simulink model "BLDC_Speed_Torque_Current_ClosedLoop"  (R2022b)
settings: Solver=ode4  StartTime=0.0  StopTime=3  FixedStep=1e-6  RelTol=1e-3
model workspace (MAT data in the model file):
  Ctrol_Mode = 4
  Current_Control_Mode = 2
  Current_PID_Upper_Limit = 1
  PWM_Period = 0.0001
  Speed_I = 10
  Speed_P = 10
  Speed_PID_Upper_Limit = 0.02
  Ts_time = 1e-06
  current_I = 10
  current_P = 100
undefined symbols (not defined in the file): DiscIntNeverNeededParam, sigbuilder_block
libraries: simulink x18, slpidlib x6, dsparch4 x3, eePwmGenerator x3, spsSeriesRLCBranchLib x2, spsPermanentMagnetSynchronousMachineLib x1, spsCurrentMeasurementLib x1, spsDCVoltageSourceLib x1, slctrlblks x1, spsTwoLevelConverterLib x1, spspowerguiLib x1
(part 1 of 2)
settings Model: Creator=31904  LastModifiedBy=31904

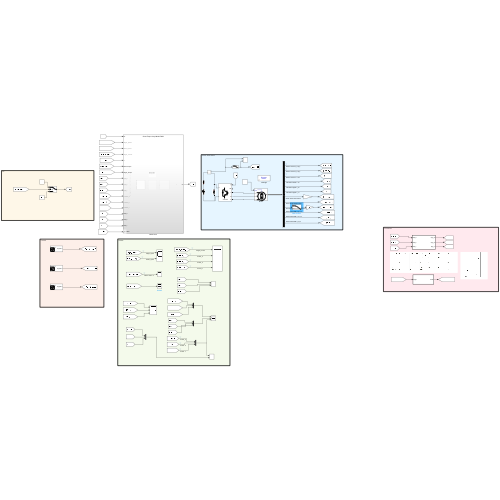
[thumbnail: Simulink's stored preview of the top-level diagram]
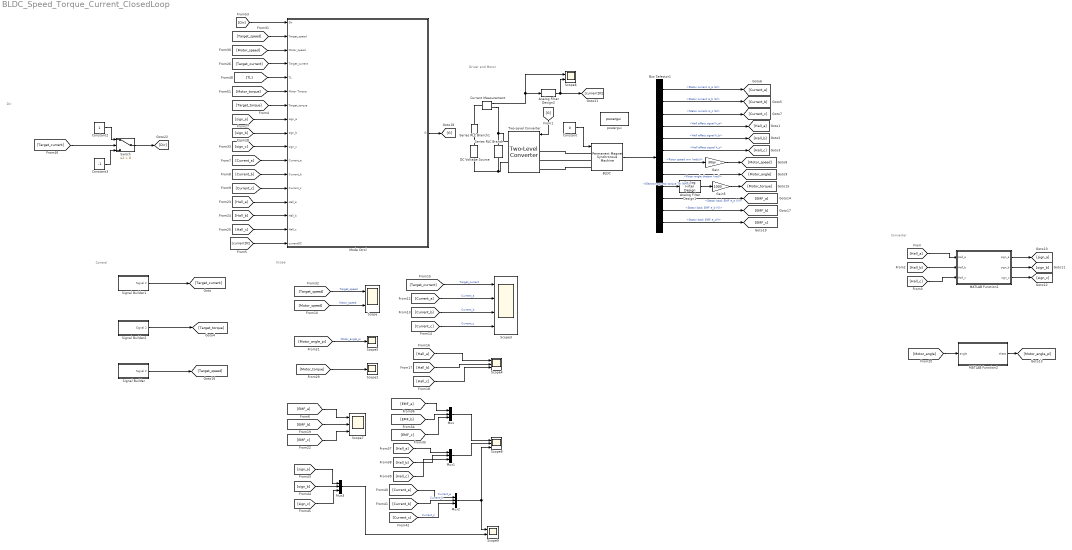
== system BLDC_Speed_Torque_Current_ClosedLoop ==
  note: Dir
  note: Converter
  note: Control
  note: Scope
  note: Driver and Motor
  Analog Filter Design1 : dsparch4/Analog Filter Design  method=Butterworth  filttype=Lowpass  N=1  Wlo=1e2  Whi=80  Rp=2  Rs=40
  Analog Filter Design2 : dsparch4/Analog Filter Design  method=Butterworth  filttype=Lowpass  N=1  Wlo=100  Whi=80  Rp=2  Rs=40
  BLDC : spsPermanentMagnetSynchronousMachineLib/Permanent Magnet Synchronous Machine  NbPhases=3  FluxDistribution=Trapezoidal  RotorType=Round  MechanicalLoad=Torque Tm  PresetModel=No  ShowDetailedParameters=on  MeasurementBus=off  Resistance=1.005  Inductance=66e-6  dqInductances=[8.5e-3,8.5e-3]  La=0.0004  MachineConstant=Torque Constant (N.m / A_peak)  Flux=0.00785  VoltageCst=3.2882  TorqueCst=0.0314  Flat=120  Mechanical=[3e-05 0 2 0]  PolePairs=4  InitialConditions=[0,0, 0,0]  InitialConditions5ph=[0 0 0 0 0 0]  RefAngle=Aligned with phase A axis (original Park)  IterativeDiscreteModel=Trapezoidal non iterative  TsBlock=-1  TsPowergui=0
  Bus Selector1 : BusSelector  OutputSignals=Stator current is_a (A),Stator current is_b (A),Stator current is_c (A),Hall effect signal h_a,Hall effect signal h_b,Hall effect signal h_c,Rotor speed wm (rad/s),Rotor angle thetam (rad),Electromagnetic torque Te (N*m),Stator back EMF e_a (V),Stator back EMF e_b (V),Stator back EMF e_cV)
  Constant : Constant  Value=0
  Constant2 : Constant
  Constant3 : Constant  Value=-1
  Current Measurement : spsCurrentMeasurementLib/Current Measurement  PhasorSimulation=off  OutputType=Complex  PSBequivalent=0
  DC Voltage Source : spsDCVoltageSourceLib/DC Voltage Source  Amplitude=28  Measurements=None
  Gain : Gain  Gain=30/pi
  Gain5 : Gain  Gain=1000
  MATLAB Function1 : MATLAB Function  TreatAsAtomicUnit=on
  MATLAB Function2 : MATLAB Function  TreatAsAtomicUnit=on
  Mode Ctrol : Subsystem  Variant=on
  Mux{,1..3} (4 alike) : Mux  Inputs=3
  Scope : Scope  NumInputPorts=2
  Scope2 : Scope
  Scope3 : Scope  NumInputPorts=4
  Scope4 : Scope  NumInputPorts=3
  Scope5 : Scope
  Scope6 : Scope  NumInputPorts=2
  Scope7 : Scope  NumInputPorts=3
  Scope8 : Scope  NumInputPorts=3
  Scope9 : Scope  NumInputPorts=2
  Series RLC Branch : spsSeriesRLCBranchLib/Series RLC Branch  LConnTagsString=__new0  RConnTagsString=__new0  BranchType=C  Resistance=1  Inductance=1e-3  SetiL0=off  InitialCurrent=0  Capacitance=1e-6  Setx0=off  InitialVoltage=0  Measurements=None
  Series RLC Branch1 : spsSeriesRLCBranchLib/Series RLC Branch  LConnTagsString=__new0  RConnTagsString=__new0  BranchType=R  Resistance=1  Inductance=1e-3  SetiL0=off  InitialCurrent=0  Capacitance=1e-6  Setx0=off  InitialVoltage=0  Measurements=None
  Signal Builder : Subsystem  Tag=STV Subsys  LoadFcn=sigbuilder_block('load');  StartFcn=sigbuilder_block('start');  StopFcn=sigbuilder_block('stop');  ClipboardFcn=sigbuilder_block('clipboard');  mask(Sigbuilder block){tuvar=[0:10]}
      mask help: Simulink:masks:SigbuilderBlock_MD
      mask init:
      | if ~strcmp(get_param(bdroot(gcbh),'SimulationStatus'),'stopped') tuvar = sigbuilder_block('maskInit'); end
      settings: CopyFcn=sigbuilder_block('copy');  DeleteFcn=sigbuilder_block('delete');  ModelCloseFcn=sigbuilder_block('modelClose');  PreSaveFcn=sigbuilder_block('preSave');  PauseFcn=sigbuilder_block('pause');  ContinueFcn=sigbuilder_block('continue');  NameChangeFcn=sigbuilder_block('namechange');  OpenFcn=sigbuilder_block('open',[281.4 79.2 550.8 400.2 ]);  CloseFcn=sigbuilder_block('close');
      mask Display: plot(0, 0, 100, 100,[2, 2, 32, 32, 2], [68, 8, 8, 68, 68],[32, 2], [38, 38], [32, 19, 2],[53, 60, 44], [32, 17, 17, 2],[16, 16, 31, 31]);txt = getActiveGroup(gcbh);text(2, 100, txt,'verticalAlignment', 'top');
  Signal Builder1 : Subsystem  Tag=STV Subsys  LoadFcn=sigbuilder_block('load');  StartFcn=sigbuilder_block('start');  StopFcn=sigbuilder_block('stop');  ClipboardFcn=sigbuilder_block('clipboard');  mask(Sigbuilder block){tuvar=[0:10]}
      mask help: Simulink:masks:SigbuilderBlock_MD
      mask init:
      | if ~strcmp(get_param(bdroot(gcbh),'SimulationStatus'),'stopped') tuvar = sigbuilder_block('maskInit'); end
      settings: CopyFcn=sigbuilder_block('copy');  DeleteFcn=sigbuilder_block('delete');  ModelCloseFcn=sigbuilder_block('modelClose');  PreSaveFcn=sigbuilder_block('preSave');  PauseFcn=sigbuilder_block('pause');  ContinueFcn=sigbuilder_block('continue');  NameChangeFcn=sigbuilder_block('namechange');  OpenFcn=sigbuilder_block('open',[5.4 30 1141.2 523.8 ]);  CloseFcn=sigbuilder_block('close');
      mask Display: plot(0, 0, 100, 100,[2, 2, 32, 32, 2], [68, 8, 8, 68, 68],[32, 2], [38, 38], [32, 19, 2],[53, 60, 44], [32, 17, 17, 2],[16, 16, 31, 31]);txt = getActiveGroup(gcbh);text(2, 100, txt,'verticalAlignment', 'top');
  Signal Builder2 : Subsystem  Tag=STV Subsys  LoadFcn=sigbuilder_block('load');  StartFcn=sigbuilder_block('start');  StopFcn=sigbuilder_block('stop');  ClipboardFcn=sigbuilder_block('clipboard');  mask(Sigbuilder block){tuvar=[0:10]}
      mask help: Simulink:masks:SigbuilderBlock_MD
      mask init:
      | if ~strcmp(get_param(bdroot(gcbh),'SimulationStatus'),'stopped') tuvar = sigbuilder_block('maskInit'); end
      settings: CopyFcn=sigbuilder_block('copy');  DeleteFcn=sigbuilder_block('delete');  ModelCloseFcn=sigbuilder_block('modelClose');  PreSaveFcn=sigbuilder_block('preSave');  PauseFcn=sigbuilder_block('pause');  ContinueFcn=sigbuilder_block('continue');  NameChangeFcn=sigbuilder_block('namechange');  OpenFcn=sigbuilder_block('open',[281.4 79.2 550.8 400.2 ]);  CloseFcn=sigbuilder_block('close');
      mask Display: plot(0, 0, 100, 100,[2, 2, 32, 32, 2], [68, 8, 8, 68, 68],[32, 2], [38, 38], [32, 19, 2],[53, 60, 44], [32, 17, 17, 2],[16, 16, 31, 31]);txt = getActiveGroup(gcbh);text(2, 100, txt,'verticalAlignment', 'top');
  Switch : Switch  Criteria=u2 > Threshold  SaturateOnIntegerOverflow=off  InputSameDT=off
  Two-Level Converter : spsTwoLevelConverterLib/Two-Level Converter  ModelType=Switching devices  Ron=0.0001  Rs=1e6  Cs=inf  Vforward=[0,0]  Ron_Diode=1e-3  Rs_Diode=1e6  Cs_Diode=inf  Vf_Diode=1e-3  Rs_CurrentSource=inf  Ron_ACsource=1e-3
  powergui : spspowerguiLib/powergui  Priority=1  SimulationMode=Discrete  SampleTime=0.000001  frequency=60  Iterations=50  frequencyindice=0  Pbase=100e6  ErrMax=1e-4  UnitsV=kV  UnitsW=MW  buscounter=0  FunctionMessages=off  echomessages=off  EnableUseOfTLC=off  CurrentSourceSwitches=off  DisableSnubberDevices=off  DisableRonSwitches=off  DisableVfSwitches=off  DisplayEquations=off  AutomaticDiscreteSolvers=off  SolverType=Tustin/Backward Euler (TBE)  Interpol=off  ExternalGateDelay=off  methode=off  Ts=100  x0status=blocks  SPID=on  SwTol=0  HookPort=off  NonlinearTolerance=1e-4  nMaxIteration=100  ContinueOnMaxIteration=off  RestoreLinks=warning  ResistiveCurrentMeasurement=off  Frange=[0:2:500]  Ylog=off  Xlog=on  ShowGrid=off  save=off  variable=ZData  structure=0  ZoomFFT=off  StartTime=0.0  cycles=1  DisplayStyle=1  fundamental=60  FreqAxis=off  MaxFrequency=1000  frequencyindicesteady=1  RmsSteady=1  display=off
  wires:
  [G] -> Two-Level Converter/1
  Bus Selector1/3 -> [Current_c]  "<Stator current is_c (A)>"
  Bus Selector1/8 -> [Motor_angle]  "<Rotor angle thetam (rad)>"
  Bus Selector1/1 -> [Current_a]  "<Stator current is_a (A)>"
  Bus Selector1/6 -> [Hall_c]  "<Hall effect signal h_c>"
  Bus Selector1/4 -> [Hall_a]  "<Hall effect signal h_a>"
  Bus Selector1/2 -> [Current_b]  "<Stator current is_b (A)>"
  Bus Selector1/7 -> Gain/1  "<Rotor speed wm (rad/s)>"
  Bus Selector1/5 -> [Hall_b]  "<Hall effect signal h_b>"
  [Hall_a] -> MATLAB Function1/1(Hall_a)
  [Hall_b] -> MATLAB Function1/2(Hall_b)
  [Hall_c] -> MATLAB Function1/3(Hall_c)
  MATLAB Function1/1(sign_a) -> [sign_a]
  MATLAB Function1/2(sign_b) -> [sign_b]
  MATLAB Function1/3(sign_c) -> [sign_c]
  [Motor_speed] -> Scope/2  "Motor_speed"
  [Current_a] -> Scope3/2  "Current_a"
  [Current_b] -> Scope3/3  "Current_b"
  [Current_c] -> Scope3/4  "Current_c"
  [Target_current] -> Scope3/1  "Target_current"
  [Hall_a] -> Scope4/1
  [Hall_b] -> Scope4/2
  [Hall_c] -> Scope4/3
  [Motor_angle] -> MATLAB Function2/1(angle)
  [Motor_angle_pi] -> Scope5/1  "Motor_angle_pi"
  MATLAB Function2/1(theta) -> [Motor_angle_pi]
  Bus Selector1/9 -> Analog Filter Design1/1  "<Electromagnetic torque Te (N*m)>"
  [Motor_torque] -> Scope2/1
  [Target_speed] -> Scope/1  "Target_speed"
  Mode Ctrol/1(G) -> [G]
  [sign_a] -> Mode Ctrol/8(sign_a)
  [sign_b] -> Mode Ctrol/9(sign_b)
  [sign_c] -> Mode Ctrol/10(sign_c)
  [Target_current] -> Mode Ctrol/4(Target_current)
  [Target_speed] -> Mode Ctrol/2(Target_speed)
  [Motor_speed] -> Mode Ctrol/3(Motor_speed)
  [Target_torque] -> Mode Ctrol/7(Target_torque)
  [Current_a] -> Mode Ctrol/11(Current_a)
  [Current_b] -> Mode Ctrol/12(Current_b)
  [Current_c] -> Mode Ctrol/13(Current_c)
  Gain/1 -> [Motor_speed]
  Bus Selector1/10 -> [EMF_a]  "<Stator back EMF e_a (V)>"
  Bus Selector1/11 -> [EMF_b]  "<Stator back EMF e_b (V)>"
  Bus Selector1/12 -> [EMF_c]  "<Stator back EMF e_cV)>"
  [EMF_a] -> Scope7/1
  [EMF_b] -> Scope7/2
  [EMF_c] -> Scope7/3
  [Hall_a] -> Mode Ctrol/14(Hall_a)
  [Hall_b] -> Mode Ctrol/15(Hall_b)
  [Hall_c] -> Mode Ctrol/16(Hall_c)
  [EMF_a] -> Mux/1
  [EMF_b] -> Mux/2
  [EMF_c] -> Mux/3
  [Hall_a] -> Mux1/1
  [Hall_b] -> Mux1/2
  [Hall_c] -> Mux1/3
  Mux1/1 -> Scope8/2
  [Current_a] -> Mux2/1  "Current_a"
  [Current_b] -> Mux2/2  "Current_b"
  [Current_c] -> Mux2/3  "Current_c"
  Mux/1 -> Scope8/1
  Mux2/1 -> Scope8/3, Scope9/1
  [sign_a] -> Mux3/1
  [sign_b] -> Mux3/2
  [sign_c] -> Mux3/3
  Mux3/1 -> Scope9/2
  BLDC/1 -> Bus Selector1/1
  [TL] -> Mode Ctrol/5(TL)
  [Motor_torque] -> Mode Ctrol/6(Motor Torque)
  Constant2/1 -> Switch/1
  Constant3/1 -> Switch/3
  Switch/1 -> [Dir]
  [Dir] -> Mode Ctrol/1(Dir)
  Gain5/1 -> [Motor_torque]
  Signal Builder/1(Signal 2) -> [Target_speed]
  Constant/1 -> BLDC/1
  Current Measurement/1 -> Scope6/1, Analog Filter Design2/1
  Analog Filter Design2/1 -> [currentDC], Scope6/2
  [currentDC] -> Mode Ctrol/17(currentDC)
  [Target_current] -> Switch/2
  Signal Builder2/1(Signal 2) -> [Target_torque]
  Signal Builder1/1(Signal 2) -> [Target_current]
  Analog Filter Design1/1 -> Gain5/1
  connections:
  DC Voltage Source/LConn1 -- Two-Level Converter/RConn2 -- Series RLC Branch/RConn1
  BLDC/LConn1 -- Two-Level Converter/LConn1
  BLDC/LConn2 -- Two-Level Converter/LConn2
  BLDC/LConn3 -- Two-Level Converter/LConn3
  Current Measurement/RConn1 -- Two-Level Converter/RConn1 -- Series RLC Branch/LConn1
  Series RLC Branch1/LConn1 -- DC Voltage Source/RConn1
  Series RLC Branch1/RConn1 -- Current Measurement/LConn1

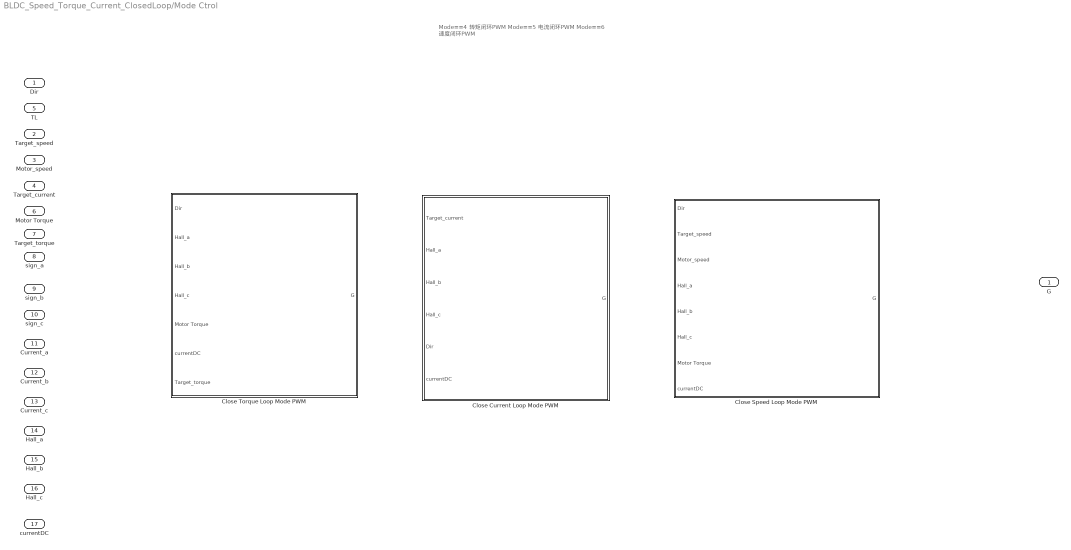
== system BLDC_Speed_Torque_Current_ClosedLoop/Mode Ctrol ==
  note: Mode==4 转矩闭环PWM
      | Mode==5 电流闭环PWM
      | Mode==6 速度闭环PWM
  Dir : Inport
  Target_speed : Inport  Port=2
  Motor_speed : Inport  Port=3
  Target_current : Inport  Port=4
  TL : Inport  Port=5
  Motor Torque : Inport  Port=6
  Target_torque : Inport  Port=7
  sign_a : Inport  Port=8
  sign_b : Inport  Port=9
  sign_c : Inport  Port=10
  Current_a : Inport  Port=11
  Current_b : Inport  Port=12
  Current_c : Inport  Port=13
  Hall_a : Inport  Port=14
  Hall_b : Inport  Port=15
  Hall_c : Inport  Port=16
  currentDC : Inport  Port=17
  Close Current Loop Mode PWM : Subsystem  TreatAsAtomicUnit=on  VariantControl=Ctrol_Mode==5
  Close Speed Loop Mode PWM : Subsystem  TreatAsAtomicUnit=on  VariantControl=Ctrol_Mode==6
  Close Torque Loop Mode PWM : Subsystem  TreatAsAtomicUnit=on  VariantControl=Ctrol_Mode==4
  G : Outport

== system BLDC_Speed_Torque_Current_ClosedLoop/Signal Builder ==
  Demux : Demux  Tag=STV Demux  Outputs=1
      settings: DisplayOption=none
  FromWs : FromWorkspace  Tag=STV FromWs  VariableName=tuvar
      SigBuilderData=|
      | common.afterFinalStr = 'Extrapolate'
      | common.sampleTime = 0
      | dataSet.timeRange = [0 10]
      | dataSet.name = 'Group 1'
      | sbobj.Groups.Name = 'Group 1'
      | sbobj.Groups.Signals.Name = 'Signal 2'
      | sbobj.Groups.Signals.XData = [0 1 1 2 2 10]
      | sbobj.Groups.Signals.YData = [1000 1000 0 0 -1000 -1000]
      | sbobj.Groups.TimeRange = [0 10]
  Signal 2 : Outport  Tag=STV Outport
  wires:
  FromWs/1 -> Demux/1
  Demux/1 -> Signal 2/1

== system BLDC_Speed_Torque_Current_ClosedLoop/Signal Builder1 ==
  Demux : Demux  Tag=STV Demux  Outputs=1
      settings: DisplayOption=none
  FromWs : FromWorkspace  Tag=STV FromWs  VariableName=tuvar
      SigBuilderData=|
      | common.afterFinalStr = 'Extrapolate'
      | common.sampleTime = 0
      | dataSet.timeRange = [0 10]
      | dataSet.name = 'Group 1'
      | sbobj.Groups.Name = 'Group 1'
      | sbobj.Groups.Signals.Name = 'Signal 2'
      | sbobj.Groups.Signals.XData = [0 1 1 2 10]
      | sbobj.Groups.Signals.YData = [0.1 0.1 -0.1 -0.1 -0.1]
      | sbobj.Groups.TimeRange = [0 10]
  Signal 2 : Outport  Tag=STV Outport
  wires:
  Demux/1 -> Signal 2/1
  FromWs/1 -> Demux/1

== system BLDC_Speed_Torque_Current_ClosedLoop/Signal Builder2 ==
  Demux : Demux  Tag=STV Demux  Outputs=1
      settings: DisplayOption=none
  FromWs : FromWorkspace  Tag=STV FromWs  VariableName=tuvar
      SigBuilderData=|
      | common.afterFinalStr = 'Extrapolate'
      | common.sampleTime = 0
      | dataSet.timeRange = [0 10]
      | dataSet.name = 'Group 1'
      | sbobj.Groups.Name = 'Group 1'
      | sbobj.Groups.Signals.Name = 'Signal 2'
      | sbobj.Groups.Signals.XData = [0 1 1 2 2 10]
      | sbobj.Groups.Signals.YData = [10 10 0 0 -10 -10]
      | sbobj.Groups.TimeRange = [0 10]
  Signal 2 : Outport  Tag=STV Outport
  wires:
  Demux/1 -> Signal 2/1
  FromWs/1 -> Demux/1

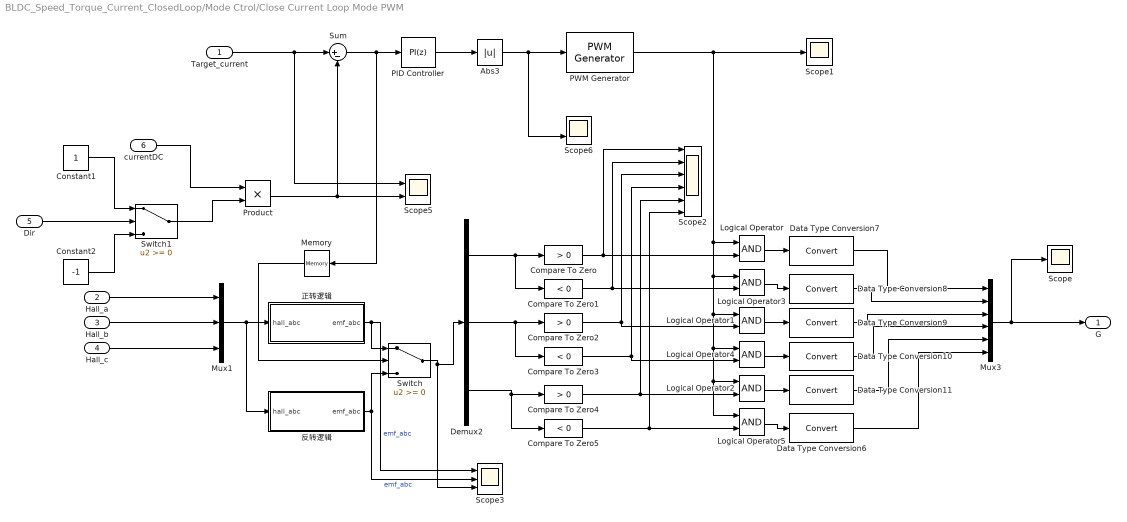
== system BLDC_Speed_Torque_Current_ClosedLoop/Mode Ctrol/Close Current Loop Mode PWM ==
  Target_current : Inport
  Hall_a : Inport  Port=2
  Hall_b : Inport  Port=3
  Hall_c : Inport  Port=4
  Dir : Inport  Port=5
  currentDC : Inport  Port=6
  Abs3 : Abs  SaturateOnIntegerOverflow=off
  Compare To Zero : simulink/Logic and Bit Operations/Compare To Zero  relop=>  OutDataTypeStr=boolean  ZeroCross=off
  Compare To Zero1 : simulink/Logic and Bit Operations/Compare To Zero  relop=<  OutDataTypeStr=boolean  ZeroCross=off
  Compare To Zero2 : simulink/Logic and Bit Operations/Compare To Zero  relop=>  OutDataTypeStr=boolean  ZeroCross=off
  Compare To Zero3 : simulink/Logic and Bit Operations/Compare To Zero  relop=<  OutDataTypeStr=boolean  ZeroCross=off
  Compare To Zero4 : simulink/Logic and Bit Operations/Compare To Zero  relop=>  OutDataTypeStr=boolean  ZeroCross=off
  Compare To Zero5 : simulink/Logic and Bit Operations/Compare To Zero  relop=<  OutDataTypeStr=boolean  ZeroCross=off
  Constant1 : Constant
  Constant2 : Constant  Value=-1
  Data Type Conversion{6..11} (6 alike) : DataTypeConversion  SaturateOnIntegerOverflow=off  RndMeth=Floor
  Demux2 : Demux  Outputs=3
  Logical Operator{,1..5} (6 alike) : Logic  AllPortsSameDT=off  OutDataTypeStr=boolean
  Memory : Memory
  Mux1 : Mux  Inputs=3
  Mux3 : Mux  Inputs=6
  PID Controller : slpidlib/PID Controller  Controller=PI  Form=Parallel  TimeDomain=Discrete-time  UseExternalTs=off  SampleTime=1e-5  IntegratorMethod=Forward Euler  FilterMethod=Forward Euler  ControllerParametersSource=internal  P=current_P  I=current_I  UseKiTs=off  D=0  N=100  UseFilter=on  TunerSelectOption=Transfer Function Based (PID Tuner App)  InitialConditionSource=internal  InitialConditionForIntegrator=0  InitialConditionForFilter=0  DifferentiatorICPrevScaledInput=0  ExternalReset=none  TrackingMode=off  Kt=1  LimitOutput=on  SatLimitsSource=internal  UpperSaturationLimit=1  LowerSaturationLimit=-1  LinearizeAsGain=off  AntiWindupMode=none  Kb=1  LimitIntegrator=on  UpperIntegratorSaturationLimit=2  LowerIntegratorSaturationLimit=-2  POutMin=[]  POutMax=[]  IOutMin=[]  IOutMax=[]  DOutMin=[]  DOutMax=[]  NOutMin=[]  NOutMax=[]  SumOutMin=[]  SumOutMax=[]  SaturationOutMin=[]  SaturationOutMax=[]  PParamMin=[]  PParamMax=[]  IParamMin=[]  IParamMax=[]  DParamMin=[]  DParamMax=[]  NParamMin=[]  NParamMax=[]  KbParamMin=[]  KbParamMax=[]  KtParamMin=[]  KtParamMax=[]  KbOutMin=[]  KbOutMax=[]  KtOutMin=[]  KtOutMax=[]  IntegratorOutMin=[]  IntegratorOutMax=[]  FilterOutMin=[]  FilterOutMax=[]  SumI1OutMin=[]  SumI1OutMax=[]  SumI2OutMin=[]  SumI2OutMax=[]  SumI3OutMin=[]  SumI3OutMax=[]  SumI4OutMin=[]  SumI4OutMax=[]  SumDOutMin=[]  SumDOutMax=[]  DifferentiatorOutMin=[]  DifferentiatorOutMax=[]  FilterDiffOutCoefMin=[]  FilterDiffOutCoefMax=[]  ReciprocalOutMin=[]  ReciprocalOutMax=[]  SumDenOutMin=[]  SumDenOutMax=[]  SumNumOutMin=[]  SumNumOutMax=[]  DivideOutMin=[]  DivideOutMax=[]  UdiffTsProdOutMin=[]  UdiffTsProdOutMax=[]  NTsProdOutMin=[]  NTsProdOutMax=[]  UintegralTsProdOutMin=[]  UintegralTsProdOutMax=[]  UngainTsProdOutMin=[]  UngainTsProdOutMax=[]  ClampingZeroOutDataTypeStr=Inherit: Inherit via back propagation  ClampingZeroOutMin=[]  ClampingZeroOutMax=[]  FilterDenConstantOutDataTypeStr=Inherit: Inherit via back propagation  FilterDenConstantOutMin=[]  FilterDenConstantOutMax=[]  PCopyOutDataTypeStr=Inherit: Inherit via back propagation  PCopyOutMin=[]  PCopyOutMax=[]  NCopyOutDataTypeStr=Inherit: Inherit via back propagation  NCopyOutMin=[]  NCopyOutMax=[]  IntegratorContinuousStateAttributes=''  IntegratorStateMustResolveToSignalObject=off  IntegratorRTWStateStorageClass=Auto  FilterContinuousStateAttributes=''  FilterStateMustResolveToSignalObject=off  FilterRTWStateStorageClass=Auto  ParallelPVariant=InternalParameters  IdealPVariant=Disabled  IVariant=InternalParameters  DVariant=Disabled  IntegratorVariant=Discrete  SatVariant=Enabled  AWVariant=Passthrough  PCopyVariant=Disabled  TRVariant=Disabled  FdbkBlocksVariant=Forward  IdealPFdbkVariant=Disabled  SatFdbkVariant=Disabled  DerivativeFilterVariant=Disabled  NVariant=Disabled  NCopyVariant=Disabled_SignalSpec  FilterICVariant=Disabled  IntegratorICVariant=InternalICs  ExternalResetVariant=Disabled  TRSumVariant=Passthrough  SumFdbkVariant=Disabled  SumVariant=Sum_PI  TsampFilterVariant=InternalTs  TsampNgainVariant=Passthrough  TsampIntegralVariant=Passthrough  ExternalSaturationOutDataTypeStr=Inherit: Same as second input
  PWM Generator : eePwmGenerator/PWM Generator  CarrCount=Up  Tper=PWM_Period  Tdelay=0  Ts=Ts_time
  Product : Product
  Scope : Scope
  Scope1 : Scope
  Scope2 : Scope  NumInputPorts=6
  Scope3 : Scope  NumInputPorts=3
  Scope5 : Scope  NumInputPorts=2
  Scope6 : Scope  NumInputPorts=2
  Sum : Sum  Inputs=|+-
  Switch : Switch  SaturateOnIntegerOverflow=off  InputSameDT=off
  Switch1 : Switch  SaturateOnIntegerOverflow=off  InputSameDT=off
  反转逻辑 : Subsystem
  正转逻辑 : Subsystem
  G : Outport
  wires:
  Target_current/1 -> Scope5/1, Sum/1
  Compare To Zero1/1 -> Logical Operator3/2, Scope2/2
  Demux2/1 -> Compare To Zero1/1, Compare To Zero/1
  Memory/1 -> Switch/2
  Data Type Conversion8/1 -> Mux3/2
  Logical Operator2/1 -> Data Type Conversion11/1
  Logical Operator3/1 -> Data Type Conversion8/1
  Compare To Zero4/1 -> Logical Operator2/2, Scope2/5
  Demux2/2 -> Compare To Zero3/1, Compare To Zero2/1
  反转逻辑/1(emf_abc) -> Scope3/2, Switch/3  "emf_abc"
  正转逻辑/1(emf_abc) -> Scope3/1, Switch/1  "emf_abc"
  Dir/1 -> Switch1/2
  Sum/1 -> Memory/1, PID Controller/1
  Data Type Conversion7/1 -> Mux3/1
  Logical Operator1/1 -> Data Type Conversion9/1
  Logical Operator5/1 -> Data Type Conversion6/1
  Logical Operator/1 -> Data Type Conversion7/1
  Hall_b/1 -> Mux1/2
  PID Controller/1 -> Abs3/1
  Mux3/1 -> Scope/1, G/1
  Mux1/1 -> 正转逻辑/1(hall_abc), 反转逻辑/1(hall_abc)
  Compare To Zero/1 -> Logical Operator/2, Scope2/1
  Switch/1 -> Scope3/3, Demux2/1
  Data Type Conversion6/1 -> Mux3/6
  Switch1/1 -> Product/2
  Logical Operator4/1 -> Data Type Conversion10/1
  Product/1 -> Scope5/2, Sum/2
  Demux2/3 -> Compare To Zero5/1, Compare To Zero4/1
  Compare To Zero5/1 -> Logical Operator5/2, Scope2/6
  PWM Generator/1 -> Logical Operator/1, Logical Operator3/1, Logical Operator1/1, Logical Operator4/1, Logical Operator5/1, Logical Operator2/1, Scope1/1
  Compare To Zero2/1 -> Logical Operator1/2, Scope2/3
  currentDC/1 -> Product/1
  Compare To Zero3/1 -> Scope2/4, Logical Operator4/2
  Hall_a/1 -> Mux1/1
  Abs3/1 -> PWM Generator/1, Scope6/2
  Data Type Conversion11/1 -> Mux3/5
  Data Type Conversion10/1 -> Mux3/4
  Constant2/1 -> Switch1/3
  Data Type Conversion9/1 -> Mux3/3
  Hall_c/1 -> Mux1/3
  Constant1/1 -> Switch1/1

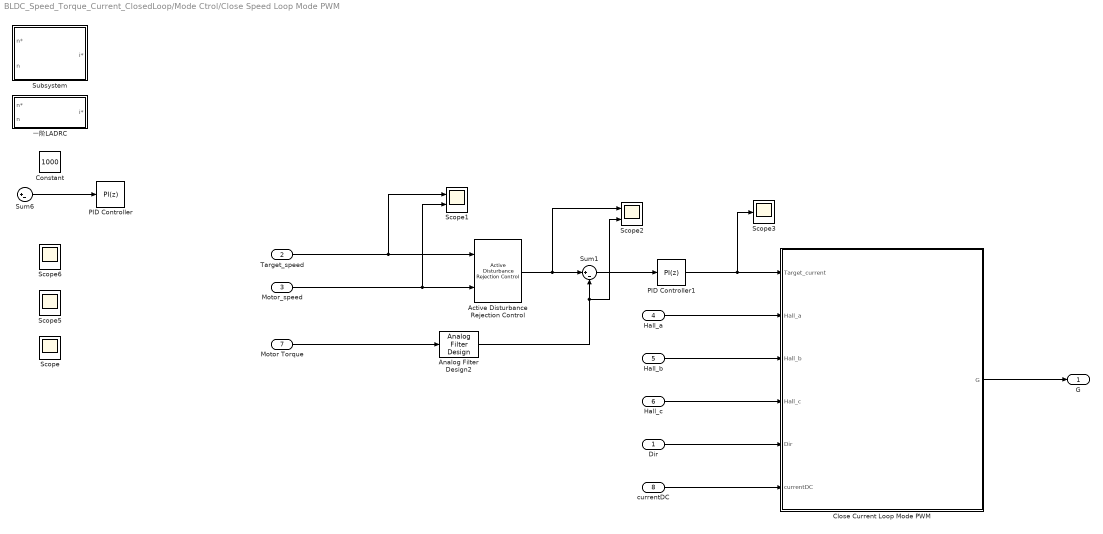
== system BLDC_Speed_Torque_Current_ClosedLoop/Mode Ctrol/Close Speed Loop Mode PWM ==
  Dir : Inport
  Target_speed : Inport  Port=2
  Motor_speed : Inport  Port=3
  Hall_a : Inport  Port=4
  Hall_b : Inport  Port=5
  Hall_c : Inport  Port=6
  Motor Torque : Inport  Port=7
  currentDC : Inport  Port=8
  Active Disturbance Rejection Control : slctrlblks/Active Disturbance Rejection Control  time_domain=discrete-time  Ts=0.00001  model_type=first-order  b0=500  wc=200  wo=1000  x0=0  ulim_checkbox=on  umax=20  umin=-20  xhat_checkbox=off
  Analog Filter Design2 : dsparch4/Analog Filter Design  method=Butterworth  filttype=Lowpass  N=1  Wlo=1e2  Whi=80  Rp=2  Rs=40
  Close Current Loop Mode PWM : Subsystem  TreatAsAtomicUnit=on  VariantControl=Ctrol_Mode==5
  Constant : Constant  Value=1000
  PID Controller : slpidlib/PID Controller  Controller=PI  Form=Parallel  TimeDomain=Discrete-time  UseExternalTs=off  SampleTime=-1  IntegratorMethod=Forward Euler  FilterMethod=Forward Euler  ControllerParametersSource=internal  P=Speed_P  I=Speed_I  UseKiTs=off  D=0  N=100  UseFilter=on  TunerSelectOption=Transfer Function Based (PID Tuner App)  InitialConditionSource=internal  InitialConditionForIntegrator=0  InitialConditionForFilter=0  DifferentiatorICPrevScaledInput=0  ExternalReset=none  TrackingMode=off  Kt=1  LimitOutput=on  SatLimitsSource=internal  UpperSaturationLimit=20  LowerSaturationLimit=-20  LinearizeAsGain=off  AntiWindupMode=none  Kb=1  LimitIntegrator=on  UpperIntegratorSaturationLimit=20  LowerIntegratorSaturationLimit=-20  POutMin=[]  POutMax=[]  IOutMin=[]  IOutMax=[]  DOutMin=[]  DOutMax=[]  NOutMin=[]  NOutMax=[]  SumOutMin=[]  SumOutMax=[]  SaturationOutMin=[]  SaturationOutMax=[]  PParamMin=[]  PParamMax=[]  IParamMin=[]  IParamMax=[]  DParamMin=[]  DParamMax=[]  NParamMin=[]  NParamMax=[]  KbParamMin=[]  KbParamMax=[]  KtParamMin=[]  KtParamMax=[]  KbOutMin=[]  KbOutMax=[]  KtOutMin=[]  KtOutMax=[]  IntegratorOutMin=[]  IntegratorOutMax=[]  FilterOutMin=[]  FilterOutMax=[]  SumI1OutMin=[]  SumI1OutMax=[]  SumI2OutMin=[]  SumI2OutMax=[]  SumI3OutMin=[]  SumI3OutMax=[]  SumI4OutMin=[]  SumI4OutMax=[]  SumDOutMin=[]  SumDOutMax=[]  DifferentiatorOutMin=[]  DifferentiatorOutMax=[]  FilterDiffOutCoefMin=[]  FilterDiffOutCoefMax=[]  ReciprocalOutMin=[]  ReciprocalOutMax=[]  SumDenOutMin=[]  SumDenOutMax=[]  SumNumOutMin=[]  SumNumOutMax=[]  DivideOutMin=[]  DivideOutMax=[]  UdiffTsProdOutMin=[]  UdiffTsProdOutMax=[]  NTsProdOutMin=[]  NTsProdOutMax=[]  UintegralTsProdOutMin=[]  UintegralTsProdOutMax=[]  UngainTsProdOutMin=[]  UngainTsProdOutMax=[]  ClampingZeroOutDataTypeStr=Inherit: Inherit via back propagation  ClampingZeroOutMin=[]  ClampingZeroOutMax=[]  FilterDenConstantOutDataTypeStr=Inherit: Inherit via back propagation  FilterDenConstantOutMin=[]  FilterDenConstantOutMax=[]  PCopyOutDataTypeStr=Inherit: Inherit via back propagation  PCopyOutMin=[]  PCopyOutMax=[]  NCopyOutDataTypeStr=Inherit: Inherit via back propagation  NCopyOutMin=[]  NCopyOutMax=[]  IntegratorContinuousStateAttributes=''  IntegratorStateMustResolveToSignalObject=off  IntegratorRTWStateStorageClass=Auto  FilterContinuousStateAttributes=''  FilterStateMustResolveToSignalObject=off  FilterRTWStateStorageClass=Auto  ParallelPVariant=InternalParameters  IdealPVariant=Disabled  IVariant=InternalParameters  DVariant=Disabled  IntegratorVariant=Discrete  SatVariant=Enabled  AWVariant=Passthrough  PCopyVariant=Disabled  TRVariant=Disabled  FdbkBlocksVariant=Forward  IdealPFdbkVariant=Disabled  SatFdbkVariant=Disabled  DerivativeFilterVariant=Disabled  NVariant=Disabled  NCopyVariant=Disabled_SignalSpec  FilterICVariant=Disabled  IntegratorICVariant=InternalICs  ExternalResetVariant=Disabled  TRSumVariant=Passthrough  SumFdbkVariant=Disabled  SumVariant=Sum_PI  TsampFilterVariant=InternalTs  TsampNgainVariant=Passthrough  TsampIntegralVariant=Passthrough  ExternalSaturationOutDataTypeStr=Inherit: Same as second input
  PID Controller1 : slpidlib/PID Controller  Controller=PI  Form=Parallel  TimeDomain=Discrete-time  UseExternalTs=off  SampleTime=-1  IntegratorMethod=Forward Euler  FilterMethod=Forward Euler  ControllerParametersSource=internal  P=50  I=10  UseKiTs=off  D=0  N=100  UseFilter=on  TunerSelectOption=Transfer Function Based (PID Tuner App)  InitialConditionSource=internal  InitialConditionForIntegrator=0  InitialConditionForFilter=0  DifferentiatorICPrevScaledInput=0  ExternalReset=none  TrackingMode=off  Kt=1  LimitOutput=on  SatLimitsSource=internal  UpperSaturationLimit=2  LowerSaturationLimit=-2  LinearizeAsGain=off  AntiWindupMode=clamping  Kb=1  LimitIntegrator=on  UpperIntegratorSaturationLimit=2  LowerIntegratorSaturationLimit=-2  POutMin=[]  POutMax=[]  IOutMin=[]  IOutMax=[]  DOutMin=[]  DOutMax=[]  NOutMin=[]  NOutMax=[]  SumOutMin=[]  SumOutMax=[]  SaturationOutMin=[]  SaturationOutMax=[]  PParamMin=[]  PParamMax=[]  IParamMin=[]  IParamMax=[]  DParamMin=[]  DParamMax=[]  NParamMin=[]  NParamMax=[]  KbParamMin=[]  KbParamMax=[]  KtParamMin=[]  KtParamMax=[]  KbOutMin=[]  KbOutMax=[]  KtOutMin=[]  KtOutMax=[]  IntegratorOutMin=[]  IntegratorOutMax=[]  FilterOutMin=[]  FilterOutMax=[]  SumI1OutMin=[]  SumI1OutMax=[]  SumI2OutMin=[]  SumI2OutMax=[]  SumI3OutMin=[]  SumI3OutMax=[]  SumI4OutMin=[]  SumI4OutMax=[]  SumDOutMin=[]  SumDOutMax=[]  DifferentiatorOutMin=[]  DifferentiatorOutMax=[]  FilterDiffOutCoefMin=[]  FilterDiffOutCoefMax=[]  ReciprocalOutMin=[]  ReciprocalOutMax=[]  SumDenOutMin=[]  SumDenOutMax=[]  SumNumOutMin=[]  SumNumOutMax=[]  DivideOutMin=[]  DivideOutMax=[]  UdiffTsProdOutMin=[]  UdiffTsProdOutMax=[]  NTsProdOutMin=[]  NTsProdOutMax=[]  UintegralTsProdOutMin=[]  UintegralTsProdOutMax=[]  UngainTsProdOutMin=[]  UngainTsProdOutMax=[]  ClampingZeroOutDataTypeStr=Inherit: Inherit via back propagation  ClampingZeroOutMin=[]  ClampingZeroOutMax=[]  FilterDenConstantOutDataTypeStr=Inherit: Inherit via back propagation  FilterDenConstantOutMin=[]  FilterDenConstantOutMax=[]  PCopyOutDataTypeStr=Inherit: Inherit via back propagation  PCopyOutMin=[]  PCopyOutMax=[]  NCopyOutDataTypeStr=Inherit: Inherit via back propagation  NCopyOutMin=[]  NCopyOutMax=[]  IntegratorContinuousStateAttributes=''  IntegratorStateMustResolveToSignalObject=off  IntegratorRTWStateStorageClass=Auto  FilterContinuousStateAttributes=''  FilterStateMustResolveToSignalObject=off  FilterRTWStateStorageClass=Auto  ParallelPVariant=InternalParameters  IdealPVariant=Disabled  IVariant=InternalParameters  DVariant=Disabled  IntegratorVariant=Discrete  SatVariant=Enabled  AWVariant=DiscClampingParallel  PCopyVariant=Disabled  TRVariant=Disabled  FdbkBlocksVariant=Forward  IdealPFdbkVariant=Disabled  SatFdbkVariant=Disabled  DerivativeFilterVariant=Disabled  NVariant=Disabled  NCopyVariant=Disabled_SignalSpec  FilterICVariant=Disabled  IntegratorICVariant=InternalICs  ExternalResetVariant=Disabled  TRSumVariant=Passthrough  SumFdbkVariant=Disabled  SumVariant=Sum_PI  TsampFilterVariant=InternalTs  TsampNgainVariant=Passthrough  TsampIntegralVariant=Passthrough  ExternalSaturationOutDataTypeStr=Inherit: Same as second input
  Scope : Scope
  Scope{1..2,5..6} (4 alike) : Scope  NumInputPorts=2
  Scope3 : Scope
  Subsystem : Subsystem
  Sum1 : Sum  Inputs=|+-
  Sum6 : Sum  Inputs=|+-
  一阶LADRC : Subsystem
  G : Outport
  wires:
  Close Current Loop Mode PWM/1(G) -> G/1
  Hall_a/1 -> Close Current Loop Mode PWM/2(Hall_a)
  Hall_b/1 -> Close Current Loop Mode PWM/3(Hall_b)
  Hall_c/1 -> Close Current Loop Mode PWM/4(Hall_c)
  Sum1/1 -> PID Controller1/1
  PID Controller1/1 -> Scope3/1, Close Current Loop Mode PWM/1(Target_current)
  Motor_speed/1 -> Scope1/2, Active Disturbance Rejection Control/2
  Dir/1 -> Close Current Loop Mode PWM/5(Dir)
  Sum6/1 -> PID Controller/1
  Motor Torque/1 -> Analog Filter Design2/1
  Analog Filter Design2/1 -> Scope2/2, Sum1/2
  currentDC/1 -> Close Current Loop Mode PWM/6(currentDC)
  Target_speed/1 -> Scope1/1, Active Disturbance Rejection Control/1
  Active Disturbance Rejection Control/1 -> Scope2/1, Sum1/1

== system BLDC_Speed_Torque_Current_ClosedLoop/Mode Ctrol/Close Torque Loop Mode PWM ==
  Dir : Inport
  Hall_a : Inport  Port=2
  Hall_b : Inport  Port=3
  Hall_c : Inport  Port=4
  Motor Torque : Inport  Port=5
  currentDC : Inport  Port=6
  Target_torque : Inport  Port=7
  Close Current Loop Mode PWM : Subsystem  TreatAsAtomicUnit=on  VariantControl=Ctrol_Mode==5
  PID Controller1 : slpidlib/PID Controller  Controller=PI  Form=Parallel  TimeDomain=Discrete-time  UseExternalTs=off  SampleTime=-1  IntegratorMethod=Forward Euler  FilterMethod=Forward Euler  ControllerParametersSource=internal  P=50  I=10  UseKiTs=off  D=0  N=100  UseFilter=on  TunerSelectOption=Transfer Function Based (PID Tuner App)  InitialConditionSource=internal  InitialConditionForIntegrator=0  InitialConditionForFilter=0  DifferentiatorICPrevScaledInput=0  ExternalReset=none  TrackingMode=off  Kt=1  LimitOutput=on  SatLimitsSource=internal  UpperSaturationLimit=2  LowerSaturationLimit=-2  LinearizeAsGain=off  AntiWindupMode=clamping  Kb=1  LimitIntegrator=off  UpperIntegratorSaturationLimit=1  LowerIntegratorSaturationLimit=-1  POutMin=[]  POutMax=[]  IOutMin=[]  IOutMax=[]  DOutMin=[]  DOutMax=[]  NOutMin=[]  NOutMax=[]  SumOutMin=[]  SumOutMax=[]  SaturationOutMin=[]  SaturationOutMax=[]  PParamMin=[]  PParamMax=[]  IParamMin=[]  IParamMax=[]  DParamMin=[]  DParamMax=[]  NParamMin=[]  NParamMax=[]  KbParamMin=[]  KbParamMax=[]  KtParamMin=[]  KtParamMax=[]  KbOutMin=[]  KbOutMax=[]  KtOutMin=[]  KtOutMax=[]  IntegratorOutMin=[]  IntegratorOutMax=[]  FilterOutMin=[]  FilterOutMax=[]  SumI1OutMin=[]  SumI1OutMax=[]  SumI2OutMin=[]  SumI2OutMax=[]  SumI3OutMin=[]  SumI3OutMax=[]  SumI4OutMin=[]  SumI4OutMax=[]  SumDOutMin=[]  SumDOutMax=[]  DifferentiatorOutMin=[]  DifferentiatorOutMax=[]  FilterDiffOutCoefMin=[]  FilterDiffOutCoefMax=[]  ReciprocalOutMin=[]  ReciprocalOutMax=[]  SumDenOutMin=[]  SumDenOutMax=[]  SumNumOutMin=[]  SumNumOutMax=[]  DivideOutMin=[]  DivideOutMax=[]  UdiffTsProdOutMin=[]  UdiffTsProdOutMax=[]  NTsProdOutMin=[]  NTsProdOutMax=[]  UintegralTsProdOutMin=[]  UintegralTsProdOutMax=[]  UngainTsProdOutMin=[]  UngainTsProdOutMax=[]  ClampingZeroOutDataTypeStr=Inherit: Inherit via back propagation  ClampingZeroOutMin=[]  ClampingZeroOutMax=[]  FilterDenConstantOutDataTypeStr=Inherit: Inherit via back propagation  FilterDenConstantOutMin=[]  FilterDenConstantOutMax=[]  PCopyOutDataTypeStr=Inherit: Inherit via back propagation  PCopyOutMin=[]  PCopyOutMax=[]  NCopyOutDataTypeStr=Inherit: Inherit via back propagation  NCopyOutMin=[]  NCopyOutMax=[]  IntegratorContinuousStateAttributes=''  IntegratorStateMustResolveToSignalObject=off  IntegratorRTWStateStorageClass=Auto  FilterContinuousStateAttributes=''  FilterStateMustResolveToSignalObject=off  FilterRTWStateStorageClass=Auto  ParallelPVariant=InternalParameters  IdealPVariant=Disabled  IVariant=InternalParameters  DVariant=Disabled  IntegratorVariant=Discrete  SatVariant=Enabled  AWVariant=DiscClampingParallel  PCopyVariant=Disabled  TRVariant=Disabled  FdbkBlocksVariant=Forward  IdealPFdbkVariant=Disabled  SatFdbkVariant=Disabled  DerivativeFilterVariant=Disabled  NVariant=Disabled  NCopyVariant=Disabled_SignalSpec  FilterICVariant=Disabled  IntegratorICVariant=InternalICs  ExternalResetVariant=Disabled  TRSumVariant=Passthrough  SumFdbkVariant=Disabled  SumVariant=Sum_PI  TsampFilterVariant=InternalTs  TsampNgainVariant=Passthrough  TsampIntegralVariant=Passthrough  ExternalSaturationOutDataTypeStr=Inherit: Same as second input
  Scope2 : Scope  NumInputPorts=2
  Scope3 : Scope
  Sum1 : Sum  Inputs=|+-
  G : Outport
  wires:
  Dir/1 -> Close Current Loop Mode PWM/5(Dir)
  Hall_c/1 -> Close Current Loop Mode PWM/4(Hall_c)
  Hall_b/1 -> Close Current Loop Mode PWM/3(Hall_b)
  Hall_a/1 -> Close Current Loop Mode PWM/2(Hall_a)
  Sum1/1 -> PID Controller1/1
  PID Controller1/1 -> Scope3/1, Close Current Loop Mode PWM/1(Target_current)
  Motor Torque/1 -> Scope2/2, Sum1/2
  currentDC/1 -> Close Current Loop Mode PWM/6(currentDC)
  Close Current Loop Mode PWM/1(G) -> G/1
  Target_torque/1 -> Scope2/1, Sum1/1

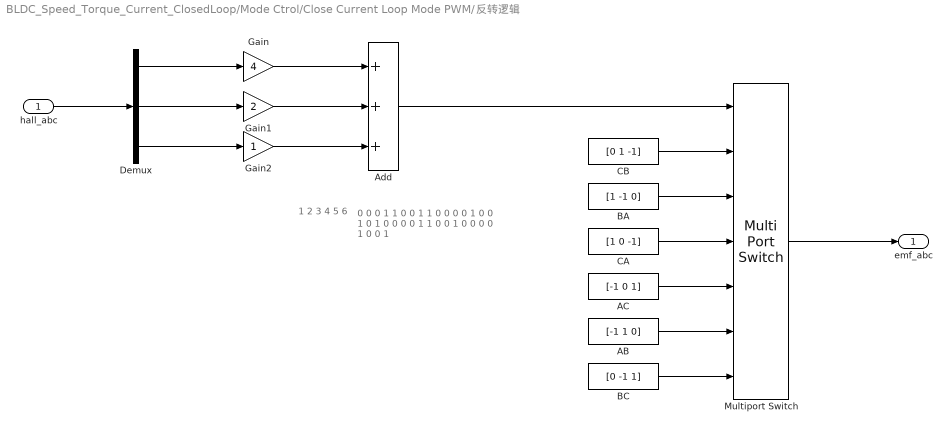
== system BLDC_Speed_Torque_Current_ClosedLoop/Mode Ctrol/Close Current Loop Mode PWM/反转逻辑 ==
  note: 0 0 0 1 1 0
      | 0 1 1 0 0 0
      | 0 1 0 0 1 0
      | 1 0 0 0 0 1
      | 1 0 0 1 0 0
      | 0 0 1 0 0 1
  note: 1
      | 2
      | 3
      | 4
      | 5
      | 6
  hall_abc : Inport
  AB : Constant  Value=[-1 1 0]
  AC : Constant  Value=[-1 0 1]
  Add : Sum  Inputs=+++
  BA : Constant  Value=[1 -1 0]
  BC : Constant  Value=[0 -1 1]
  CA : Constant  Value=[1 0 -1]
  CB : Constant  Value=[0 1 -1]
  Demux : Demux  Outputs=3
  Gain : Gain  Gain=4
  Gain1 : Gain  Gain=2
  Gain2 : Gain
  Multiport Switch : MultiPortSwitch  Inputs=6  DiagnosticForDefault=None  SaturateOnIntegerOverflow=off  InputSameDT=off
  emf_abc : Outport
  wires:
  BA/1 -> Multiport Switch/3
  CB/1 -> Multiport Switch/2
  CA/1 -> Multiport Switch/4
  AB/1 -> Multiport Switch/6
  BC/1 -> Multiport Switch/7
  Multiport Switch/1 -> emf_abc/1
  Add/1 -> Multiport Switch/1
  AC/1 -> Multiport Switch/5
  Gain/1 -> Add/1
  Gain1/1 -> Add/2
  Gain2/1 -> Add/3
  Demux/2 -> Gain1/1
  Demux/1 -> Gain/1
  Demux/3 -> Gain2/1
  hall_abc/1 -> Demux/1

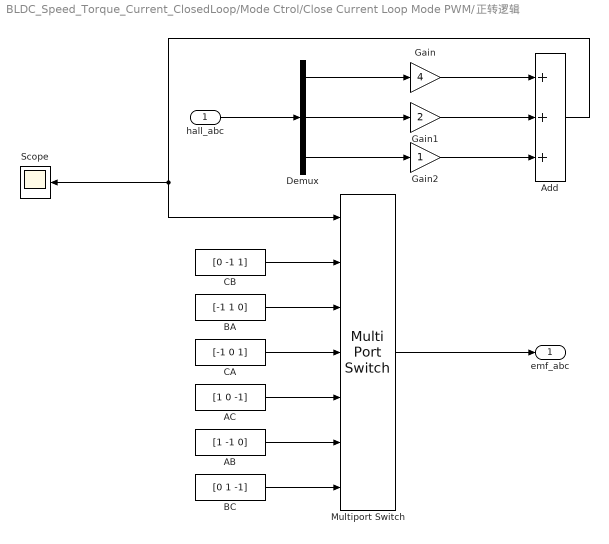
== system BLDC_Speed_Torque_Current_ClosedLoop/Mode Ctrol/Close Current Loop Mode PWM/正转逻辑 ==
  hall_abc : Inport
  AB : Constant  Value=[1 -1 0]
  AC : Constant  Value=[1 0 -1]
  Add : Sum  Inputs=+++
  BA : Constant  Value=[-1 1 0]
  BC : Constant  Value=[0 1 -1]
  CA : Constant  Value=[-1 0 1]
  CB : Constant  Value=[0 -1 1]
  Demux : Demux  Outputs=3
  Gain : Gain  Gain=4
  Gain1 : Gain  Gain=2
  Gain2 : Gain
  Multiport Switch : MultiPortSwitch  Inputs=6  DiagnosticForDefault=None  SaturateOnIntegerOverflow=off  InputSameDT=off
  Scope : Scope
  emf_abc : Outport
  wires:
  BA/1 -> Multiport Switch/3
  CB/1 -> Multiport Switch/2
  CA/1 -> Multiport Switch/4
  AB/1 -> Multiport Switch/6
  BC/1 -> Multiport Switch/7
  Multiport Switch/1 -> emf_abc/1
  Add/1 -> Scope/1, Multiport Switch/1
  AC/1 -> Multiport Switch/5
  Gain/1 -> Add/1
  Gain1/1 -> Add/2
  Gain2/1 -> Add/3
  Demux/2 -> Gain1/1
  Demux/1 -> Gain/1
  Demux/3 -> Gain2/1
  hall_abc/1 -> Demux/1

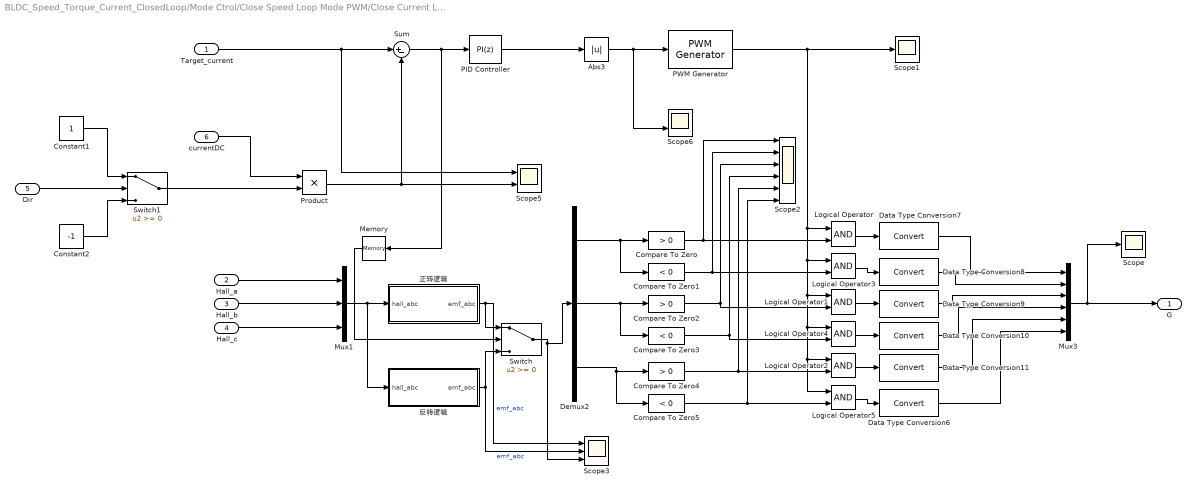
== system BLDC_Speed_Torque_Current_ClosedLoop/Mode Ctrol/Close Speed Loop Mode PWM/Close Current Loop Mode PWM ==
  Target_current : Inport
  Hall_a : Inport  Port=2
  Hall_b : Inport  Port=3
  Hall_c : Inport  Port=4
  Dir : Inport  Port=5
  currentDC : Inport  Port=6
  Abs3 : Abs  SaturateOnIntegerOverflow=off
  Compare To Zero : simulink/Logic and Bit Operations/Compare To Zero  relop=>  OutDataTypeStr=boolean  ZeroCross=off
  Compare To Zero1 : simulink/Logic and Bit Operations/Compare To Zero  relop=<  OutDataTypeStr=boolean  ZeroCross=off
  Compare To Zero2 : simulink/Logic and Bit Operations/Compare To Zero  relop=>  OutDataTypeStr=boolean  ZeroCross=off
  Compare To Zero3 : simulink/Logic and Bit Operations/Compare To Zero  relop=<  OutDataTypeStr=boolean  ZeroCross=off
  Compare To Zero4 : simulink/Logic and Bit Operations/Compare To Zero  relop=>  OutDataTypeStr=boolean  ZeroCross=off
  Compare To Zero5 : simulink/Logic and Bit Operations/Compare To Zero  relop=<  OutDataTypeStr=boolean  ZeroCross=off
  Constant1 : Constant
  Constant2 : Constant  Value=-1
  Data Type Conversion{6..11} (6 alike) : DataTypeConversion  SaturateOnIntegerOverflow=off  RndMeth=Floor
  Demux2 : Demux  Outputs=3
  Logical Operator{,1..5} (6 alike) : Logic  AllPortsSameDT=off  OutDataTypeStr=boolean
  Memory : Memory
  Mux1 : Mux  Inputs=3
  Mux3 : Mux  Inputs=6
  PID Controller : slpidlib/PID Controller  Controller=PI  Form=Parallel  TimeDomain=Discrete-time  UseExternalTs=off  SampleTime=1e-5  IntegratorMethod=Forward Euler  FilterMethod=Forward Euler  ControllerParametersSource=internal  P=current_P  I=current_I  UseKiTs=off  D=0  N=100  UseFilter=on  TunerSelectOption=Transfer Function Based (PID Tuner App)  InitialConditionSource=internal  InitialConditionForIntegrator=0  InitialConditionForFilter=0  DifferentiatorICPrevScaledInput=0  ExternalReset=none  TrackingMode=off  Kt=1  LimitOutput=on  SatLimitsSource=internal  UpperSaturationLimit=1  LowerSaturationLimit=-1  LinearizeAsGain=off  AntiWindupMode=none  Kb=1  LimitIntegrator=on  UpperIntegratorSaturationLimit=2  LowerIntegratorSaturationLimit=-2  POutMin=[]  POutMax=[]  IOutMin=[]  IOutMax=[]  DOutMin=[]  DOutMax=[]  NOutMin=[]  NOutMax=[]  SumOutMin=[]  SumOutMax=[]  SaturationOutMin=[]  SaturationOutMax=[]  PParamMin=[]  PParamMax=[]  IParamMin=[]  IParamMax=[]  DParamMin=[]  DParamMax=[]  NParamMin=[]  NParamMax=[]  KbParamMin=[]  KbParamMax=[]  KtParamMin=[]  KtParamMax=[]  KbOutMin=[]  KbOutMax=[]  KtOutMin=[]  KtOutMax=[]  IntegratorOutMin=[]  IntegratorOutMax=[]  FilterOutMin=[]  FilterOutMax=[]  SumI1OutMin=[]  SumI1OutMax=[]  SumI2OutMin=[]  SumI2OutMax=[]  SumI3OutMin=[]  SumI3OutMax=[]  SumI4OutMin=[]  SumI4OutMax=[]  SumDOutMin=[]  SumDOutMax=[]  DifferentiatorOutMin=[]  DifferentiatorOutMax=[]  FilterDiffOutCoefMin=[]  FilterDiffOutCoefMax=[]  ReciprocalOutMin=[]  ReciprocalOutMax=[]  SumDenOutMin=[]  SumDenOutMax=[]  SumNumOutMin=[]  SumNumOutMax=[]  DivideOutMin=[]  DivideOutMax=[]  UdiffTsProdOutMin=[]  UdiffTsProdOutMax=[]  NTsProdOutMin=[]  NTsProdOutMax=[]  UintegralTsProdOutMin=[]  UintegralTsProdOutMax=[]  UngainTsProdOutMin=[]  UngainTsProdOutMax=[]  ClampingZeroOutDataTypeStr=Inherit: Inherit via back propagation  ClampingZeroOutMin=[]  ClampingZeroOutMax=[]  FilterDenConstantOutDataTypeStr=Inherit: Inherit via back propagation  FilterDenConstantOutMin=[]  FilterDenConstantOutMax=[]  PCopyOutDataTypeStr=Inherit: Inherit via back propagation  PCopyOutMin=[]  PCopyOutMax=[]  NCopyOutDataTypeStr=Inherit: Inherit via back propagation  NCopyOutMin=[]  NCopyOutMax=[]  IntegratorContinuousStateAttributes=''  IntegratorStateMustResolveToSignalObject=off  IntegratorRTWStateStorageClass=Auto  FilterContinuousStateAttributes=''  FilterStateMustResolveToSignalObject=off  FilterRTWStateStorageClass=Auto  ParallelPVariant=InternalParameters  IdealPVariant=Disabled  IVariant=InternalParameters  DVariant=Disabled  IntegratorVariant=Discrete  SatVariant=Enabled  AWVariant=Passthrough  PCopyVariant=Disabled  TRVariant=Disabled  FdbkBlocksVariant=Forward  IdealPFdbkVariant=Disabled  SatFdbkVariant=Disabled  DerivativeFilterVariant=Disabled  NVariant=Disabled  NCopyVariant=Disabled_SignalSpec  FilterICVariant=Disabled  IntegratorICVariant=InternalICs  ExternalResetVariant=Disabled  TRSumVariant=Passthrough  SumFdbkVariant=Disabled  SumVariant=Sum_PI  TsampFilterVariant=InternalTs  TsampNgainVariant=Passthrough  TsampIntegralVariant=Passthrough  ExternalSaturationOutDataTypeStr=Inherit: Same as second input
  PWM Generator : eePwmGenerator/PWM Generator  CarrCount=Up  Tper=PWM_Period  Tdelay=0  Ts=Ts_time
  Product : Product
  Scope : Scope
  Scope1 : Scope
  Scope2 : Scope  NumInputPorts=6
  Scope3 : Scope  NumInputPorts=3
  Scope5 : Scope  NumInputPorts=2
  Scope6 : Scope  NumInputPorts=2
  Sum : Sum  Inputs=|+-
  Switch : Switch  SaturateOnIntegerOverflow=off  InputSameDT=off
  Switch1 : Switch  SaturateOnIntegerOverflow=off  InputSameDT=off
  反转逻辑 : Subsystem
  正转逻辑 : Subsystem
  G : Outport
  wires:
  Target_current/1 -> Scope5/1, Sum/1
  Compare To Zero1/1 -> Logical Operator3/2, Scope2/2
  Demux2/1 -> Compare To Zero1/1, Compare To Zero/1
  Memory/1 -> Switch/2
  Data Type Conversion8/1 -> Mux3/2
  Logical Operator2/1 -> Data Type Conversion11/1
  Logical Operator3/1 -> Data Type Conversion8/1
  Compare To Zero4/1 -> Logical Operator2/2, Scope2/5
  Demux2/2 -> Compare To Zero3/1, Compare To Zero2/1
  反转逻辑/1(emf_abc) -> Scope3/2, Switch/3  "emf_abc"
  正转逻辑/1(emf_abc) -> Scope3/1, Switch/1  "emf_abc"
  Dir/1 -> Switch1/2
  Sum/1 -> Memory/1, PID Controller/1
  Data Type Conversion7/1 -> Mux3/1
  Logical Operator1/1 -> Data Type Conversion9/1
  Logical Operator5/1 -> Data Type Conversion6/1
  Logical Operator/1 -> Data Type Conversion7/1
  Hall_b/1 -> Mux1/2
  PID Controller/1 -> Abs3/1
  Mux3/1 -> Scope/1, G/1
  Mux1/1 -> 正转逻辑/1(hall_abc), 反转逻辑/1(hall_abc)
  Compare To Zero/1 -> Logical Operator/2, Scope2/1
  Switch/1 -> Scope3/3, Demux2/1
  Data Type Conversion6/1 -> Mux3/6
  Switch1/1 -> Product/2
  Logical Operator4/1 -> Data Type Conversion10/1
  Product/1 -> Scope5/2, Sum/2
  Demux2/3 -> Compare To Zero5/1, Compare To Zero4/1
  Compare To Zero5/1 -> Logical Operator5/2, Scope2/6
  PWM Generator/1 -> Logical Operator/1, Logical Operator3/1, Logical Operator1/1, Logical Operator4/1, Logical Operator5/1, Logical Operator2/1, Scope1/1
  Compare To Zero2/1 -> Logical Operator1/2, Scope2/3
  currentDC/1 -> Product/1
  Compare To Zero3/1 -> Scope2/4, Logical Operator4/2
  Hall_a/1 -> Mux1/1
  Abs3/1 -> PWM Generator/1, Scope6/2
  Data Type Conversion11/1 -> Mux3/5
  Data Type Conversion10/1 -> Mux3/4
  Constant2/1 -> Switch1/3
  Data Type Conversion9/1 -> Mux3/3
  Hall_c/1 -> Mux1/3
  Constant1/1 -> Switch1/1

== system BLDC_Speed_Torque_Current_ClosedLoop/Mode Ctrol/Close Speed Loop Mode PWM/Subsystem ==
  n* : Inport
  n : Inport  Port=2
  Saturation : Saturate  UpperLimit=30  LowerLimit=-30
  Scope : Scope  NumInputPorts=2
  Scope1 : Scope
  Subsystem2 : Subsystem
  TD : Subsystem
  nlsef : Subsystem
  i* : Outport
  wires:
  nlsef/1(ut) -> Scope/1, Saturation/1, Subsystem2/1(ut)
  Saturation/1 -> Scope/2, i*/1
  n/1 -> Subsystem2/2(n)
  Subsystem2/2(z22) -> nlsef/2(z22)
  Subsystem2/1(z21) -> nlsef/3(z21)
  TD/1(z11) -> Scope1/1, nlsef/1(z11)
  n*/1 -> TD/1(n*)

== system BLDC_Speed_Torque_Current_ClosedLoop/Mode Ctrol/Close Speed Loop Mode PWM/一阶LADRC ==
  n* : Inport
  n : Inport  Port=2
  1/b : Gain  Gain=1/350
  ESO : Subsystem
  Memory : Memory
  Memory1 : Memory
  Saturation : Saturate  UpperLimit=20  LowerLimit=-20
  Sum : Sum  Inputs=|+-
  Sum1 : Sum  Inputs=|+-
  b : Gain  Gain=350
  wc=w0/4 : Gain
  i* : Outport
  wires:
  n*/1 -> Sum/1
  Sum/1 -> wc=w0/4/1
  wc=w0/4/1 -> Sum1/1
  Sum1/1 -> i*/1, Saturation/1, b/1
  b/1 -> ESO/1(ut)
  n/1 -> ESO/2(n)
  ESO/2(z2) -> 1/b/1
  1/b/1 -> Memory/1
  ESO/1(z1) -> Memory1/1
  Memory/1 -> Sum1/2
  Memory1/1 -> Sum/2

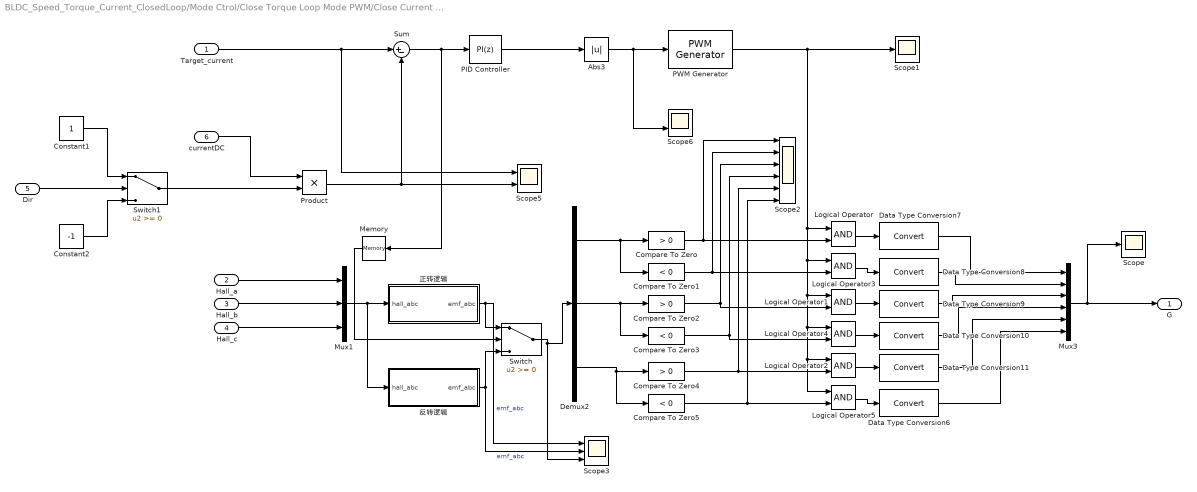
== system BLDC_Speed_Torque_Current_ClosedLoop/Mode Ctrol/Close Torque Loop Mode PWM/Close Current Loop Mode PWM ==
  Target_current : Inport
  Hall_a : Inport  Port=2
  Hall_b : Inport  Port=3
  Hall_c : Inport  Port=4
  Dir : Inport  Port=5
  currentDC : Inport  Port=6
  Abs3 : Abs  SaturateOnIntegerOverflow=off
  Compare To Zero : simulink/Logic and Bit Operations/Compare To Zero  relop=>  OutDataTypeStr=boolean  ZeroCross=off
  Compare To Zero1 : simulink/Logic and Bit Operations/Compare To Zero  relop=<  OutDataTypeStr=boolean  ZeroCross=off
  Compare To Zero2 : simulink/Logic and Bit Operations/Compare To Zero  relop=>  OutDataTypeStr=boolean  ZeroCross=off
  Compare To Zero3 : simulink/Logic and Bit Operations/Compare To Zero  relop=<  OutDataTypeStr=boolean  ZeroCross=off
  Compare To Zero4 : simulink/Logic and Bit Operations/Compare To Zero  relop=>  OutDataTypeStr=boolean  ZeroCross=off
  Compare To Zero5 : simulink/Logic and Bit Operations/Compare To Zero  relop=<  OutDataTypeStr=boolean  ZeroCross=off
  Constant1 : Constant
  Constant2 : Constant  Value=-1
  Data Type Conversion{6..11} (6 alike) : DataTypeConversion  SaturateOnIntegerOverflow=off  RndMeth=Floor
  Demux2 : Demux  Outputs=3
  Logical Operator{,1..5} (6 alike) : Logic  AllPortsSameDT=off  OutDataTypeStr=boolean
  Memory : Memory
  Mux1 : Mux  Inputs=3
  Mux3 : Mux  Inputs=6
  PID Controller : slpidlib/PID Controller  Controller=PI  Form=Parallel  TimeDomain=Discrete-time  UseExternalTs=off  SampleTime=1e-5  IntegratorMethod=Forward Euler  FilterMethod=Forward Euler  ControllerParametersSource=internal  P=current_P  I=current_I  UseKiTs=off  D=0  N=100  UseFilter=on  TunerSelectOption=Transfer Function Based (PID Tuner App)  InitialConditionSource=internal  InitialConditionForIntegrator=0  InitialConditionForFilter=0  DifferentiatorICPrevScaledInput=0  ExternalReset=none  TrackingMode=off  Kt=1  LimitOutput=on  SatLimitsSource=internal  UpperSaturationLimit=1  LowerSaturationLimit=-1  LinearizeAsGain=off  AntiWindupMode=none  Kb=1  LimitIntegrator=on  UpperIntegratorSaturationLimit=2  LowerIntegratorSaturationLimit=-2  POutMin=[]  POutMax=[]  IOutMin=[]  IOutMax=[]  DOutMin=[]  DOutMax=[]  NOutMin=[]  NOutMax=[]  SumOutMin=[]  SumOutMax=[]  SaturationOutMin=[]  SaturationOutMax=[]  PParamMin=[]  PParamMax=[]  IParamMin=[]  IParamMax=[]  DParamMin=[]  DParamMax=[]  NParamMin=[]  NParamMax=[]  KbParamMin=[]  KbParamMax=[]  KtParamMin=[]  KtParamMax=[]  KbOutMin=[]  KbOutMax=[]  KtOutMin=[]  KtOutMax=[]  IntegratorOutMin=[]  IntegratorOutMax=[]  FilterOutMin=[]  FilterOutMax=[]  SumI1OutMin=[]  SumI1OutMax=[]  SumI2OutMin=[]  SumI2OutMax=[]  SumI3OutMin=[]  SumI3OutMax=[]  SumI4OutMin=[]  SumI4OutMax=[]  SumDOutMin=[]  SumDOutMax=[]  DifferentiatorOutMin=[]  DifferentiatorOutMax=[]  FilterDiffOutCoefMin=[]  FilterDiffOutCoefMax=[]  ReciprocalOutMin=[]  ReciprocalOutMax=[]  SumDenOutMin=[]  SumDenOutMax=[]  SumNumOutMin=[]  SumNumOutMax=[]  DivideOutMin=[]  DivideOutMax=[]  UdiffTsProdOutMin=[]  UdiffTsProdOutMax=[]  NTsProdOutMin=[]  NTsProdOutMax=[]  UintegralTsProdOutMin=[]  UintegralTsProdOutMax=[]  UngainTsProdOutMin=[]  UngainTsProdOutMax=[]  ClampingZeroOutDataTypeStr=Inherit: Inherit via back propagation  ClampingZeroOutMin=[]  ClampingZeroOutMax=[]  FilterDenConstantOutDataTypeStr=Inherit: Inherit via back propagation  FilterDenConstantOutMin=[]  FilterDenConstantOutMax=[]  PCopyOutDataTypeStr=Inherit: Inherit via back propagation  PCopyOutMin=[]  PCopyOutMax=[]  NCopyOutDataTypeStr=Inherit: Inherit via back propagation  NCopyOutMin=[]  NCopyOutMax=[]  IntegratorContinuousStateAttributes=''  IntegratorStateMustResolveToSignalObject=off  IntegratorRTWStateStorageClass=Auto  FilterContinuousStateAttributes=''  FilterStateMustResolveToSignalObject=off  FilterRTWStateStorageClass=Auto  ParallelPVariant=InternalParameters  IdealPVariant=Disabled  IVariant=InternalParameters  DVariant=Disabled  IntegratorVariant=Discrete  SatVariant=Enabled  AWVariant=Passthrough  PCopyVariant=Disabled  TRVariant=Disabled  FdbkBlocksVariant=Forward  IdealPFdbkVariant=Disabled  SatFdbkVariant=Disabled  DerivativeFilterVariant=Disabled  NVariant=Disabled  NCopyVariant=Disabled_SignalSpec  FilterICVariant=Disabled  IntegratorICVariant=InternalICs  ExternalResetVariant=Disabled  TRSumVariant=Passthrough  SumFdbkVariant=Disabled  SumVariant=Sum_PI  TsampFilterVariant=InternalTs  TsampNgainVariant=Passthrough  TsampIntegralVariant=Passthrough  ExternalSaturationOutDataTypeStr=Inherit: Same as second input
  PWM Generator : eePwmGenerator/PWM Generator  CarrCount=Up  Tper=PWM_Period  Tdelay=0  Ts=Ts_time
  Product : Product
  Scope : Scope
  Scope1 : Scope
  Scope2 : Scope  NumInputPorts=6
  Scope3 : Scope  NumInputPorts=3
  Scope5 : Scope  NumInputPorts=2
  Scope6 : Scope  NumInputPorts=2
  Sum : Sum  Inputs=|+-
  Switch : Switch  SaturateOnIntegerOverflow=off  InputSameDT=off
  Switch1 : Switch  SaturateOnIntegerOverflow=off  InputSameDT=off
  反转逻辑 : Subsystem
  正转逻辑 : Subsystem
  G : Outport
  wires:
  Data Type Conversion11/1 -> Mux3/5
  Dir/1 -> Switch1/2
  Data Type Conversion9/1 -> Mux3/3
  Hall_c/1 -> Mux1/3
  反转逻辑/1(emf_abc) -> Scope3/2, Switch/3  "emf_abc"
  Product/1 -> Scope5/2, Sum/2
  Memory/1 -> Switch/2
  currentDC/1 -> Product/1
  Hall_a/1 -> Mux1/1
  Logical Operator5/1 -> Data Type Conversion6/1
  Compare To Zero4/1 -> Logical Operator2/2, Scope2/5
  Constant1/1 -> Switch1/1
  Hall_b/1 -> Mux1/2
  Compare To Zero3/1 -> Scope2/4, Logical Operator4/2
  Constant2/1 -> Switch1/3
  Logical Operator4/1 -> Data Type Conversion10/1
  Compare To Zero5/1 -> Logical Operator5/2, Scope2/6
  Sum/1 -> Memory/1, PID Controller/1
  PWM Generator/1 -> Logical Operator/1, Logical Operator3/1, Logical Operator1/1, Logical Operator4/1, Logical Operator5/1, Logical Operator2/1, Scope1/1
  Abs3/1 -> PWM Generator/1, Scope6/2
  Compare To Zero2/1 -> Logical Operator1/2, Scope2/3
  Mux3/1 -> Scope/1, G/1
  Logical Operator1/1 -> Data Type Conversion9/1
  Data Type Conversion7/1 -> Mux3/1
  Data Type Conversion6/1 -> Mux3/6
  Switch/1 -> Scope3/3, Demux2/1
  Compare To Zero/1 -> Logical Operator/2, Scope2/1
  正转逻辑/1(emf_abc) -> Scope3/1, Switch/1  "emf_abc"
  Mux1/1 -> 正转逻辑/1(hall_abc), 反转逻辑/1(hall_abc)
  Compare To Zero1/1 -> Logical Operator3/2, Scope2/2
  PID Controller/1 -> Abs3/1
  Logical Operator/1 -> Data Type Conversion7/1
  Demux2/3 -> Compare To Zero5/1, Compare To Zero4/1
  Logical Operator3/1 -> Data Type Conversion8/1
  Logical Operator2/1 -> Data Type Conversion11/1
  Data Type Conversion10/1 -> Mux3/4
  Switch1/1 -> Product/2
  Demux2/2 -> Compare To Zero3/1, Compare To Zero2/1
  Data Type Conversion8/1 -> Mux3/2
  Demux2/1 -> Compare To Zero1/1, Compare To Zero/1
  Target_current/1 -> Scope5/1, Sum/1
